simulink model "FFCharacteristicBySize"  (Simulink 9.2)
settings: Solver=ode45  StartTime=0.0  StopTime=1  RelTol=1e-3  EnableMultiTasking=on
libraries: NeuroModelerLibrary x20, simulink x9
settings Model: Creator=Bakhshiev  LastModifiedBy=Bakhshiev
settings OptimizationCC: ExpressionDepthLimit=2147483647
settings DebuggingCC: SolverPrmCheckMsg=warning

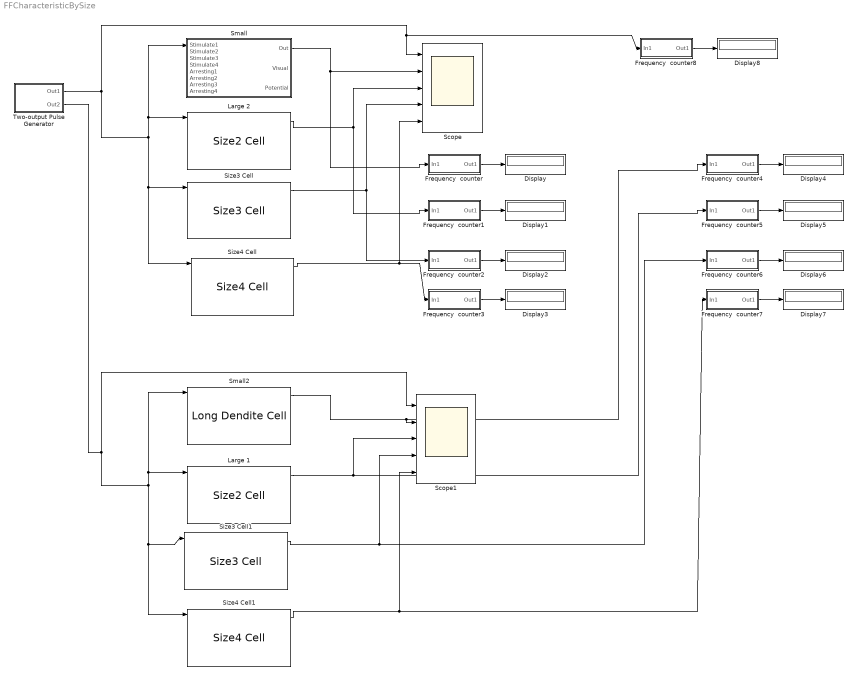
== system FFCharacteristicBySize ==
  Display{,1..8} (9 alike) : Display
  Frequency  counter : Subsystem
  Frequency  counter1 : Subsystem
  Frequency  counter2 : Subsystem
  Frequency  counter3 : Subsystem
  Frequency  counter4 : Subsystem
  Frequency  counter5 : Subsystem
  Frequency  counter6 : Subsystem
  Frequency  counter7 : Subsystem
  Frequency  counter8 : Subsystem
  Large 1 : NeuroModelerLibrary/Sized Cells/Size2 Cell  SystemSampleTime=-1
      link override Synapse: PSMode=1
  Large 2 : NeuroModelerLibrary/Sized Cells/Size2 Cell  SystemSampleTime=-1
  Scope : Scope  NumInputPorts=5
  Scope1 : Scope  NumInputPorts=5
  Size3 Cell : NeuroModelerLibrary/Sized Cells/Size3 Cell  SystemSampleTime=-1
  Size3 Cell1 : NeuroModelerLibrary/Sized Cells/Size3 Cell  SystemSampleTime=-1
      link override Synapse2: PSMode=1
  Size4 Cell : NeuroModelerLibrary/Sized Cells/Size4 Cell  SystemSampleTime=-1
  Size4 Cell1 : NeuroModelerLibrary/Sized Cells/Size4 Cell  SystemSampleTime=-1
      link override Synapse: PSMode=1
  Small : Subsystem  AncestorBlock=NeuroModelerLibrary/Dendrites Cells/Long Dendite Cell
  Small2 : NeuroModelerLibrary/Dendrites Cells/Long Dendite Cell  SystemSampleTime=-1
      link override Synapse: PSMode=1
  Two-output Pulse Generator : Subsystem  mask{A=1, P1=50, P2=2, PW=1, ST=0.001, OOn1=0.00, OOff1=0.5, OOn2=0.0, OOff2=1}
      mask prompts: A "Amplitude"; P1 "Out1: Period (number of samples)"; P2 "Out2: Period (number of samples)"; PW "Pulse Width (number of samples)"; ST "Sample Time"; OOn1 "Out1 On (seconds)"; OOff1 "Out1 Off (seconds)"; OOn2 "Out2 On (seconds)"; OOff2 "Out2 Off (seconds)"
  wires:
  Two-output Pulse Generator/1(Out1) -> Small/1(Stimulate1), Large 2/1, Size3 Cell/1, Size4 Cell/1, Scope/1, Frequency  counter8/1(In1)
  Small/1(Out) -> Frequency  counter/1(In1), Scope/2
  Large 2/1 -> Frequency  counter1/1(In1), Scope/3
  Size4 Cell/1 -> Scope/5, Frequency  counter3/1(In1)
  Frequency  counter/1(Out1) -> Display/1
  Frequency  counter1/1(Out1) -> Display1/1
  Frequency  counter2/1(Out1) -> Display2/1
  Frequency  counter3/1(Out1) -> Display3/1
  Two-output Pulse Generator/2(Out2) -> Small2/1, Large 1/1, Size3 Cell1/1, Size4 Cell1/1, Scope1/1
  Small2/1 -> Frequency  counter4/1(In1), Scope1/2
  Large 1/1 -> Frequency  counter5/1(In1), Scope1/3
  Size4 Cell1/1 -> Scope1/5, Frequency  counter7/1(In1)
  Size3 Cell1/1 -> Scope1/4, Frequency  counter6/1(In1)
  Frequency  counter4/1(Out1) -> Display4/1
  Frequency  counter5/1(Out1) -> Display5/1
  Frequency  counter6/1(Out1) -> Display6/1
  Frequency  counter7/1(Out1) -> Display7/1
  Frequency  counter8/1(Out1) -> Display8/1
  Size3 Cell/1 -> Scope/4, Frequency  counter2/1(In1)

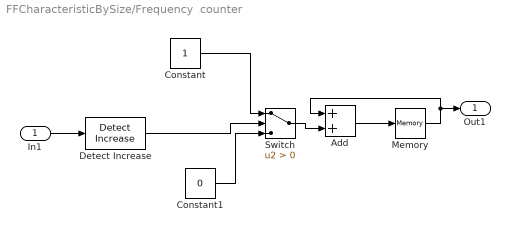
== system FFCharacteristicBySize/Frequency  counter ==
  In1 : Inport
  Add : Sum
  Constant : Constant
  Constant1 : Constant  Value=0
  Detect Increase : simulink/Logic and Bit Operations/Detect Increase  vinit=0.0  OutDataTypeStr=uint8
  Memory : Memory
  Switch : Switch  Criteria=u2 > Threshold
  Out1 : Outport
  wires:
  Detect Increase/1 -> Switch/2
  Constant1/1 -> Switch/3
  Constant/1 -> Switch/1
  Switch/1 -> Add/2
  Add/1 -> Memory/1
  Memory/1 -> Add/1, Out1/1
  In1/1 -> Detect Increase/1

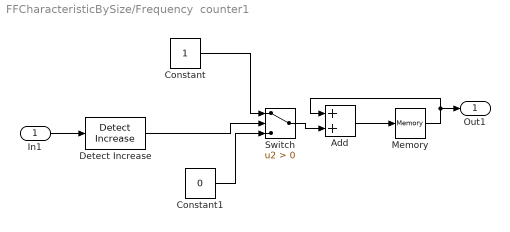
== system FFCharacteristicBySize/Frequency  counter1 ==
  In1 : Inport
  Add : Sum
  Constant : Constant
  Constant1 : Constant  Value=0
  Detect Increase : simulink/Logic and Bit Operations/Detect Increase  vinit=0.0  OutDataTypeStr=uint8
  Memory : Memory
  Switch : Switch  Criteria=u2 > Threshold
  Out1 : Outport
  wires:
  Detect Increase/1 -> Switch/2
  Constant1/1 -> Switch/3
  Constant/1 -> Switch/1
  Switch/1 -> Add/2
  Add/1 -> Memory/1
  Memory/1 -> Add/1, Out1/1
  In1/1 -> Detect Increase/1

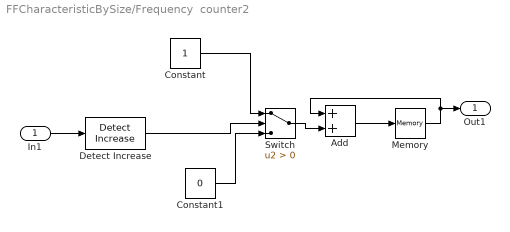
== system FFCharacteristicBySize/Frequency  counter2 ==
  In1 : Inport
  Add : Sum
  Constant : Constant
  Constant1 : Constant  Value=0
  Detect Increase : simulink/Logic and Bit Operations/Detect Increase  vinit=0.0  OutDataTypeStr=uint8
  Memory : Memory
  Switch : Switch  Criteria=u2 > Threshold
  Out1 : Outport
  wires:
  Detect Increase/1 -> Switch/2
  Constant1/1 -> Switch/3
  Constant/1 -> Switch/1
  Switch/1 -> Add/2
  Add/1 -> Memory/1
  Memory/1 -> Add/1, Out1/1
  In1/1 -> Detect Increase/1

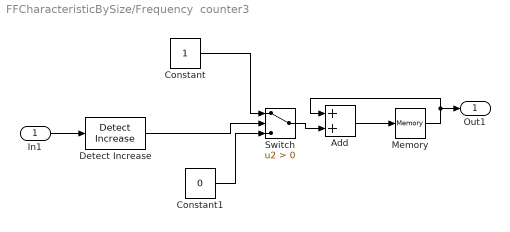
== system FFCharacteristicBySize/Frequency  counter3 ==
  In1 : Inport
  Add : Sum
  Constant : Constant
  Constant1 : Constant  Value=0
  Detect Increase : simulink/Logic and Bit Operations/Detect Increase  vinit=0.0  OutDataTypeStr=uint8
  Memory : Memory
  Switch : Switch  Criteria=u2 > Threshold
  Out1 : Outport
  wires:
  Detect Increase/1 -> Switch/2
  Constant1/1 -> Switch/3
  Constant/1 -> Switch/1
  Switch/1 -> Add/2
  Add/1 -> Memory/1
  Memory/1 -> Add/1, Out1/1
  In1/1 -> Detect Increase/1

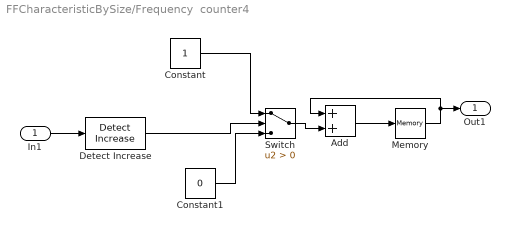
== system FFCharacteristicBySize/Frequency  counter4 ==
  In1 : Inport
  Add : Sum
  Constant : Constant
  Constant1 : Constant  Value=0
  Detect Increase : simulink/Logic and Bit Operations/Detect Increase  vinit=0.0  OutDataTypeStr=uint8
  Memory : Memory
  Switch : Switch  Criteria=u2 > Threshold
  Out1 : Outport
  wires:
  Detect Increase/1 -> Switch/2
  Constant1/1 -> Switch/3
  Constant/1 -> Switch/1
  Switch/1 -> Add/2
  Add/1 -> Memory/1
  Memory/1 -> Add/1, Out1/1
  In1/1 -> Detect Increase/1

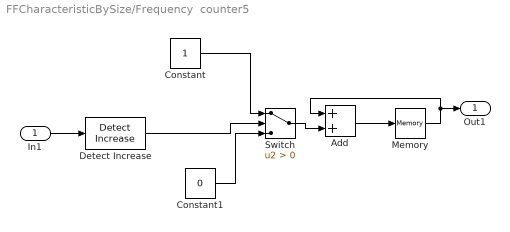
== system FFCharacteristicBySize/Frequency  counter5 ==
  In1 : Inport
  Add : Sum
  Constant : Constant
  Constant1 : Constant  Value=0
  Detect Increase : simulink/Logic and Bit Operations/Detect Increase  vinit=0.0  OutDataTypeStr=uint8
  Memory : Memory
  Switch : Switch  Criteria=u2 > Threshold
  Out1 : Outport
  wires:
  Detect Increase/1 -> Switch/2
  Constant1/1 -> Switch/3
  Constant/1 -> Switch/1
  Switch/1 -> Add/2
  Add/1 -> Memory/1
  Memory/1 -> Add/1, Out1/1
  In1/1 -> Detect Increase/1

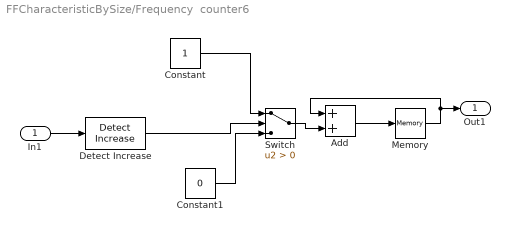
== system FFCharacteristicBySize/Frequency  counter6 ==
  In1 : Inport
  Add : Sum
  Constant : Constant
  Constant1 : Constant  Value=0
  Detect Increase : simulink/Logic and Bit Operations/Detect Increase  vinit=0.0  OutDataTypeStr=uint8
  Memory : Memory
  Switch : Switch  Criteria=u2 > Threshold
  Out1 : Outport
  wires:
  Detect Increase/1 -> Switch/2
  Constant1/1 -> Switch/3
  Constant/1 -> Switch/1
  Switch/1 -> Add/2
  Add/1 -> Memory/1
  Memory/1 -> Add/1, Out1/1
  In1/1 -> Detect Increase/1

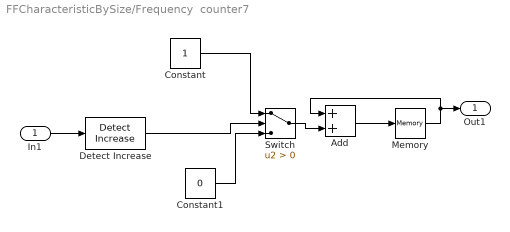
== system FFCharacteristicBySize/Frequency  counter7 ==
  In1 : Inport
  Add : Sum
  Constant : Constant
  Constant1 : Constant  Value=0
  Detect Increase : simulink/Logic and Bit Operations/Detect Increase  vinit=0.0  OutDataTypeStr=uint8
  Memory : Memory
  Switch : Switch  Criteria=u2 > Threshold
  Out1 : Outport
  wires:
  Detect Increase/1 -> Switch/2
  Constant1/1 -> Switch/3
  Constant/1 -> Switch/1
  Switch/1 -> Add/2
  Add/1 -> Memory/1
  Memory/1 -> Add/1, Out1/1
  In1/1 -> Detect Increase/1

== system FFCharacteristicBySize/Frequency  counter8 ==
  In1 : Inport
  Add : Sum
  Constant : Constant
  Constant1 : Constant  Value=0
  Detect Increase : simulink/Logic and Bit Operations/Detect Increase  vinit=0.0  OutDataTypeStr=uint8
  Memory : Memory
  Switch : Switch  Criteria=u2 > Threshold
  Out1 : Outport
  wires:
  Detect Increase/1 -> Switch/2
  Constant1/1 -> Switch/3
  Constant/1 -> Switch/1
  Switch/1 -> Add/2
  Add/1 -> Memory/1
  Memory/1 -> Add/1, Out1/1
  In1/1 -> Detect Increase/1

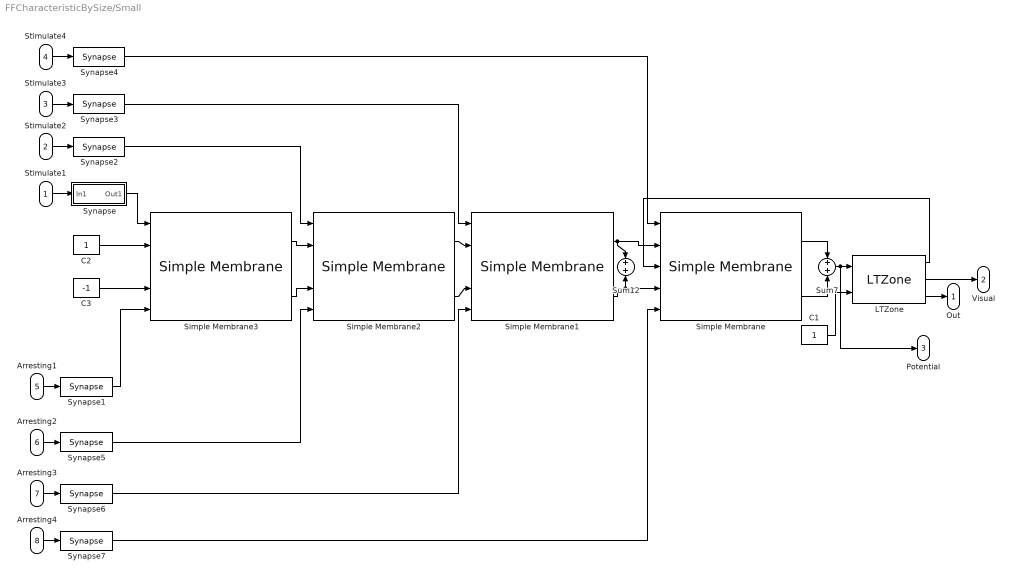
== system FFCharacteristicBySize/Small ==
  Stimulate1 : Inport
  Stimulate2 : Inport  Port=2
  Stimulate3 : Inport  Port=3
  Stimulate4 : Inport  Port=4
  Arresting1 : Inport  Port=5
  Arresting2 : Inport  Port=6
  Arresting3 : Inport  Port=7
  Arresting4 : Inport  Port=8
  C1 : Constant
  C2 : Constant
  C3 : Constant  Value=-1
  LTZone : NeuroModelerLibrary/Neuron Elements/LTZone  NM=1  FB=1.7  IT=0.005  T=0.001
  Simple Membrane{,1..3} (4 alike) : NeuroModelerLibrary/Neuron Elements/Simple Membrane  ACm=1e-9  ARm=1e7  ECm=1e-9  ERm=1e7  ARFm=1e8  ERFm=1e8
  Sum12 : Sum  SaturateOnIntegerOverflow=on  InputSameDT=on  OutDataTypeStr=Inherit: Same as first input
  Sum7 : Sum  SaturateOnIntegerOverflow=on  InputSameDT=on  OutDataTypeStr=Inherit: Same as first input
  Synapse : Subsystem  mask{SecretionTC=0.001, DecompositionTC=0.01, ksi=2, gamma=1e8, PSMode=0}
      mask prompts: SecretionTC "Mediator Secretion"; DecompositionTC "Mediator Decomposition"; PSMode "Presynaptic Mode"
  Synapse{1..7} (7 alike) : NeuroModelerLibrary/Neuron Elements/Synapse  SecretionTC=0.001  DecompositionTC=0.01  UseKsi=on  ksi=2  gamma=1e8
  Out : Outport
  Visual : Outport  Port=2
  Potential : Outport  Port=3
  wires:
  Synapse7/1 -> Simple Membrane/5
  Arresting4/1 -> Synapse7/1
  Synapse6/1 -> Simple Membrane1/5
  Arresting3/1 -> Synapse6/1
  Synapse5/1 -> Simple Membrane2/5
  Arresting2/1 -> Synapse5/1
  Stimulate4/1 -> Synapse4/1
  Synapse4/1 -> Simple Membrane/1
  Stimulate3/1 -> Synapse3/1
  Synapse3/1 -> Simple Membrane1/1
  Stimulate2/1 -> Synapse2/1
  Synapse2/1 -> Simple Membrane2/1
  Synapse/1(Out1) -> Simple Membrane3/1
  C2/1 -> Simple Membrane3/2
  C3/1 -> Simple Membrane3/4
  Synapse1/1 -> Simple Membrane3/5
  Simple Membrane3/2 -> Simple Membrane2/4
  Simple Membrane3/1 -> Simple Membrane2/2
  Simple Membrane2/2 -> Simple Membrane1/4
  Simple Membrane2/1 -> Simple Membrane1/2
  LTZone/2 -> Visual/1
  LTZone/3 -> Out/1
  C1/1 -> LTZone/2
  Stimulate1/1 -> Synapse/1(In1)
  Arresting1/1 -> Synapse1/1
  Simple Membrane1/1 -> Simple Membrane/2, Sum12/1
  Simple Membrane1/2 -> Simple Membrane/4, Sum12/2
  Sum7/1 -> LTZone/1, Potential/1
  LTZone/1 -> Simple Membrane/3
  Simple Membrane/1 -> Sum7/1
  Simple Membrane/2 -> Sum7/2

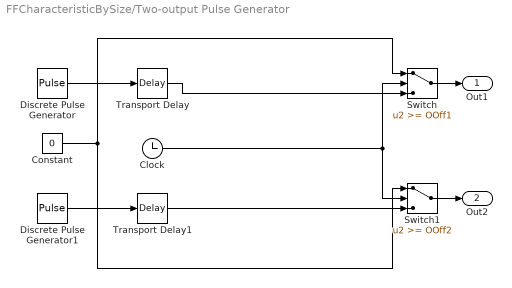
== system FFCharacteristicBySize/Two-output Pulse Generator ==
  Clock : Clock
  Constant : Constant  Value=0
  Discrete Pulse Generator : DiscretePulseGenerator  Amplitude=A  Period=P1  PulseWidth=PW  SampleTime=ST
  Discrete Pulse Generator1 : DiscretePulseGenerator  Amplitude=A  Period=P2  PulseWidth=PW  SampleTime=ST
  Switch : Switch  Threshold=OOff1  SaturateOnIntegerOverflow=on  InputSameDT=on
  Switch1 : Switch  Threshold=OOff2  SaturateOnIntegerOverflow=on  InputSameDT=on
  Transport Delay : TransportDelay  DelayTime=OOn1
  Transport Delay1 : TransportDelay  DelayTime=OOn2
  Out1 : Outport  InitialOutput=0
  Out2 : Outport  Port=2  InitialOutput=0
  wires:
  Discrete Pulse Generator/1 -> Transport Delay/1
  Constant/1 -> Switch/1, Switch1/1
  Discrete Pulse Generator1/1 -> Transport Delay1/1
  Transport Delay1/1 -> Switch1/3
  Transport Delay/1 -> Switch/3
  Clock/1 -> Switch/2, Switch1/2
  Switch/1 -> Out1/1
  Switch1/1 -> Out2/1

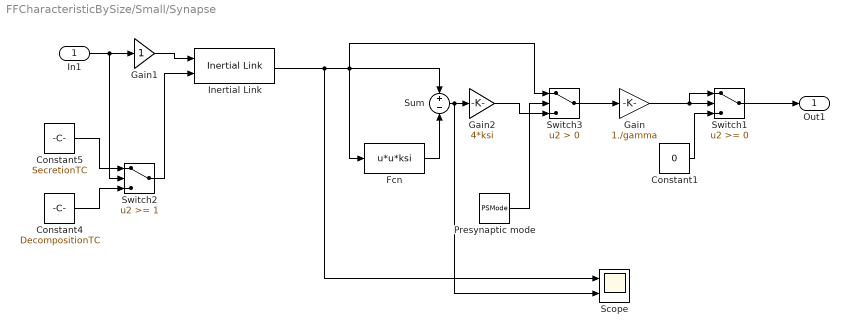
== system FFCharacteristicBySize/Small/Synapse ==
  In1 : Inport
  Constant1 : Constant  Value=0
  Constant4 : Constant  Value=DecompositionTC
  Constant5 : Constant  Value=SecretionTC
  Fcn : Fcn  Expr=u*u*ksi
  Gain : Gain  Gain=1./gamma  SaturateOnIntegerOverflow=on  OutDataTypeStr=Inherit: Same as input  ParamDataTypeStr=Inherit: Same as input
  Gain1 : Gain  SaturateOnIntegerOverflow=on  OutDataTypeStr=Inherit: Same as input  ParamDataTypeStr=Inherit: Same as input
  Gain2 : Gain  Gain=4*ksi  SaturateOnIntegerOverflow=on  OutDataTypeStr=Inherit: Same as input  ParamDataTypeStr=Inherit: Same as input
  Inertial Link : NeuroModelerLibrary/Support/Inertial Link  SystemSampleTime=-1
  Presynaptic mode : Constant  Value=PSMode
  Scope : Scope  NumInputPorts=2
  Sum : Sum  Inputs=+-  SaturateOnIntegerOverflow=on
  Switch1 : Switch
  Switch2 : Switch  Threshold=1
  Switch3 : Switch  Criteria=u2 > Threshold
  Out1 : Outport
  wires:
  Gain2/1 -> Switch3/3
  Presynaptic mode/1 -> Switch3/2
  Switch3/1 -> Gain/1
  Switch1/1 -> Out1/1
  Gain1/1 -> Inertial Link/1
  Constant1/1 -> Switch1/3
  Gain/1 -> Switch1/1, Switch1/2
  Switch2/1 -> Inertial Link/2
  Constant5/1 -> Switch2/1
  Constant4/1 -> Switch2/3
  Inertial Link/1 -> Scope/1, Sum/1, Fcn/1, Switch3/1
  Sum/1 -> Scope/2, Gain2/1
  In1/1 -> Gain1/1, Switch2/2
  Fcn/1 -> Sum/2
